simulink library "vehicle_cl"  (R2018b)
settings: Solver=VariableStepAuto  StartTime=0.0  StopTime=10.0  RelTol=1e-3
undefined symbols (not defined in the file): initializeVariantsFromBlock, sim_param, simParam
libraries: vehicle000_cl x1, vehicle001_cl x1, AyazOctLiftingBdy_cl x1, eulAng2RotMat_ul x1, thrAttachPtKinematics_ul x1
settings Model: Creator=mcobb  LastModifiedBy=mcobb

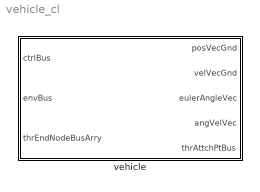
== system vehicle_cl ==
  vehicle : Subsystem  LoadFcn=initializeVariantsFromBlock(gcb)  InitFcn=initializeVariantsFromBlock(gcb)  StartFcn=initializeVariantsFromBlock(gcb)  Variant=on
      settings: PreSaveFcn=initializeVariantsFromBlock(gcb)

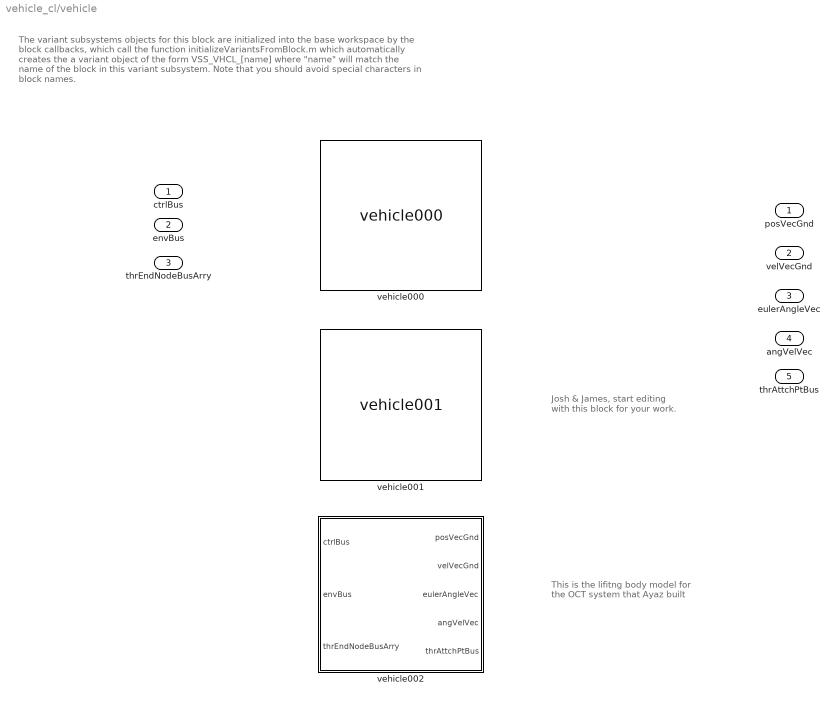
== system vehicle_cl/vehicle ==
  note: This is the lifitng body model for the OCT system that Ayaz built
  note: Josh & James, start editing
      | with this block for your work.
  note: The variant subsystems objects for this block are initialized into the base
      | workspace by the block callbacks, which call the function initializeVariantsFromBlock.m
      | which automatically creates the a variant object of the form
      | VSS_VHCL_[name]
      | where "name" will match the name of the block in this variant subsystem.
      | Note that you should avoid special characters in block names.
  ctrlBus : Inport  OutDataTypeStr=Bus: ctrlBus
  envBus : Inport  Port=2  OutDataTypeStr=Bus: envBus
  thrEndNodeBusArry : Inport  Port=3
  vehicle000 : vehicle000_cl/vehicle000  VariantControl=VSS_VHCL_vehicle000  m=simParam.geom_param.mass.Value  inertiaMatrix=simParam.geom_param.MI.Value  initPos=simParam.initPosVec.Value  initVel=simParam.initVelVec.Value  initEulerAngles=simParam.initEulAng.Value  initAngVel=simParam.initPltAngVel.Value  rho=simParam.env_param.density.Value  vol=simParam.geom_param.vol.Value  grav=simParam.env_param.grav.Value  thrAttchStruct=lftBdyMmtArms  CB2CMVec=simParam.geom_param.center_of_buoy.Value  turb1Pos=simParam.turbine_param.R1turb_cm.Value  turb2Pos=simParam.turbine_param.R2turb_cm.Value  turbDiam=simParam.turbine_param.d_turbine.Value  turbCp=simParam.turbine_param.Cp_turb.Value  turbCd=simParam.turbine_param.CD_turb.Value  CLTable=CLtot_2D_Tbl  CDTable=CDtot_2D_Tbl  CMxTable=Cltot_2D_Tbl  CMyTable=Cmtot_2D_Tbl  CMzTable=Cntot_2D_Tbl  CS_gain=k_CS_gain  SRef=simParam.avlSRef.Value  BRef=simParam.avlBRef.Value  CRef=simParam.avlCRef.Value
  vehicle001 : vehicle001_cl/vehicle001  VariantControl=VSS_VHCL_vehicle001  m=1  inertiaMatrix=eye(3)  initPos=[0 0 0]  initVel=[0 0 0]  initEulerAngles=[0 0 0]  initAngVel=[0 0 0]  rho=1.225  vol=1  grav=9.81  thrAttchStruct=lftBdyMmtArms  CB2CMVec=[1 0 0]  turb1Pos=0  turb2Pos=0  turbDiam=0  turbCp=0  turbCd=0  CLTable=CLtotTbl  CDTable=CLtotTbl  CMxTable=CLtotTbl  CMyTable=CLtotTbl  CMzTable=CLtotTbl  CS_gain=CS_gain  SRef=CLtotTbl  BRef=CLtotTbl  CRef=CLtotTbl
  vehicle002 : Subsystem  VariantControl=VSS_VHCL_vehicle002
      mask init:
      | load('OrginalOCctModelVars');
  posVecGnd : Outport
  velVecGnd : Outport  Port=2
  eulerAngleVec : Outport  Port=3
  angVelVec : Outport  Port=4
  thrAttchPtBus : Outport  Port=5

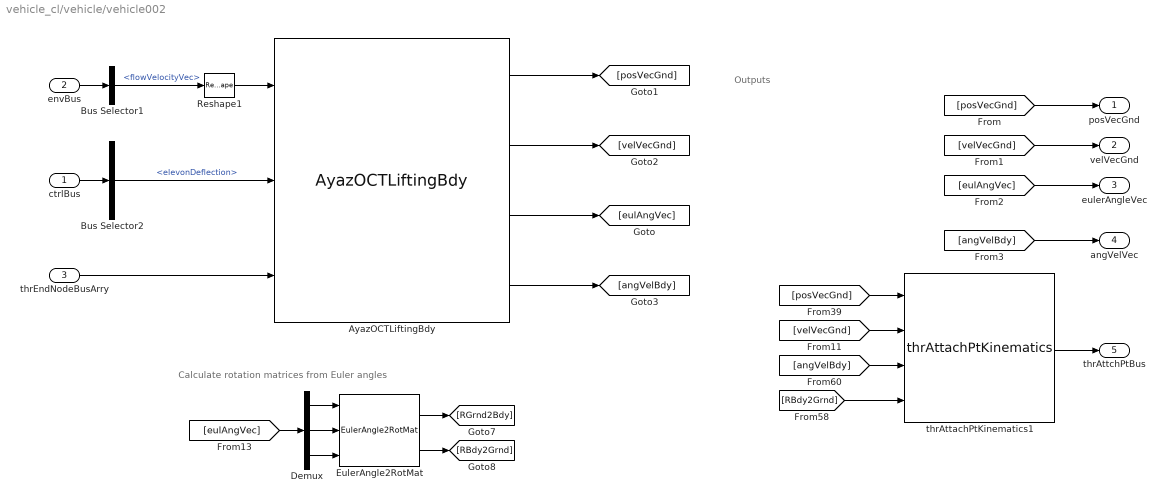
== system vehicle_cl/vehicle/vehicle002 ==
  note: Outputs
  note: Calculate rotation matrices from Euler angles
  ctrlBus : Inport  OutDataTypeStr=Bus: ctrlBus
  envBus : Inport  Port=2  OutDataTypeStr=Bus: envBus
  thrEndNodeBusArry : Inport  Port=3
  AyazOCTLiftingBdy : AyazOctLiftingBdy_cl/AyazOCTLiftingBdy  sim_param=sim_param  initCon=origOCT_iniCon
  Bus Selector1 : BusSelector  OutputSignals=flowVelocityVec
  Bus Selector2 : BusSelector  OutputSignals=elevonDeflection
  Demux : Demux  Outputs=3
  EulerAngle2RotMat : eulAng2RotMat_ul/EulerAngle2RotMat  SystemSampleTime=-1
  Reshape1 : Reshape  OutputDimensionality=Column vector (2-D)
  thrAttachPtKinematics1 : thrAttachPtKinematics_ul/thrAttachPtKinematics  atchPts=[sim_param.tether_imp_nodes.R1n_cm,sim_param.tether_imp_nodes.R2n_cm,sim_param.tether_imp_nodes.R3n_cm]
  posVecGnd : Outport
  velVecGnd : Outport  Port=2
  eulerAngleVec : Outport  Port=3
  angVelVec : Outport  Port=4
  thrAttchPtBus : Outport  Port=5
  wires:
  Bus Selector1/1 -> Reshape1/1  "<flowVelocityVec>"
  Reshape1/1 -> AyazOCTLiftingBdy/1
  envBus/1 -> Bus Selector1/1
  ctrlBus/1 -> Bus Selector2/1
  Bus Selector2/1 -> AyazOCTLiftingBdy/2  "<elevonDeflection>"
  thrEndNodeBusArry/1 -> AyazOCTLiftingBdy/3
  [posVecGnd] -> thrAttachPtKinematics1/1
  [RBdy2Grnd] -> thrAttachPtKinematics1/4
  thrAttachPtKinematics1/1 -> thrAttchPtBus/1
  [angVelBdy] -> thrAttachPtKinematics1/3
  [velVecGnd] -> thrAttachPtKinematics1/2
  Demux/3 -> EulerAngle2RotMat/3
  [eulAngVec] -> Demux/1
  Demux/2 -> EulerAngle2RotMat/2
  Demux/1 -> EulerAngle2RotMat/1
  EulerAngle2RotMat/1 -> [RGrnd2Bdy]
  EulerAngle2RotMat/2 -> [RBdy2Grnd]
  AyazOCTLiftingBdy/3 -> [eulAngVec]
  AyazOCTLiftingBdy/1 -> [posVecGnd]
  AyazOCTLiftingBdy/2 -> [velVecGnd]
  AyazOCTLiftingBdy/4 -> [angVelBdy]
  [posVecGnd] -> posVecGnd/1
  [velVecGnd] -> velVecGnd/1
  [eulAngVec] -> eulerAngleVec/1
  [angVelBdy] -> angVelVec/1
